simulink model "dashboard_boilerplate"  (R2018b)
settings: Solver=FixedStepDiscrete  StartTime=0.0  StopTime=40  FixedStep=1e-3  RelTol=1e-3
settings Model: EnablePacing=on  Creator=kjartan  LastModifiedBy=kjartan

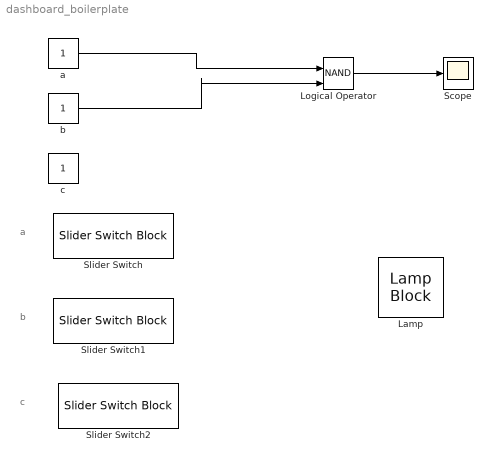
== system dashboard_boilerplate ==
  note: a
  note: b
  note: c
  Lamp : LampBlock  WebBlockId=4
  Logical Operator : Logic  Operator=NAND  IconShape=distinctive  AllPortsSameDT=off  OutDataTypeStr=boolean
  Scope : Scope
  Slider Switch : SliderSwitchBlock  WebBlockId=2
      settings: Values={{'Off', 'On'}, [0 1]}
  Slider Switch1 : SliderSwitchBlock  WebBlockId=14
      settings: Values={{'Off', 'On'}, [0 1]}
  Slider Switch2 : SliderSwitchBlock  WebBlockId=15
      settings: Values={{'Off', 'On'}, [0 1]}
  a : Constant
  b : Constant
  c : Constant
  wires:
  Logical Operator/1 -> Scope/1
  a/1 -> Logical Operator/1
  b/1 -> Logical Operator/2
